simulink model "ex3"  (R2020a)
settings: Solver=VariableStepAuto  StartTime=0.0  StopTime=10.0  RelTol=1e-3
settings Model: Creator=Kundan Patil  LastModifiedBy=Kundan Patil

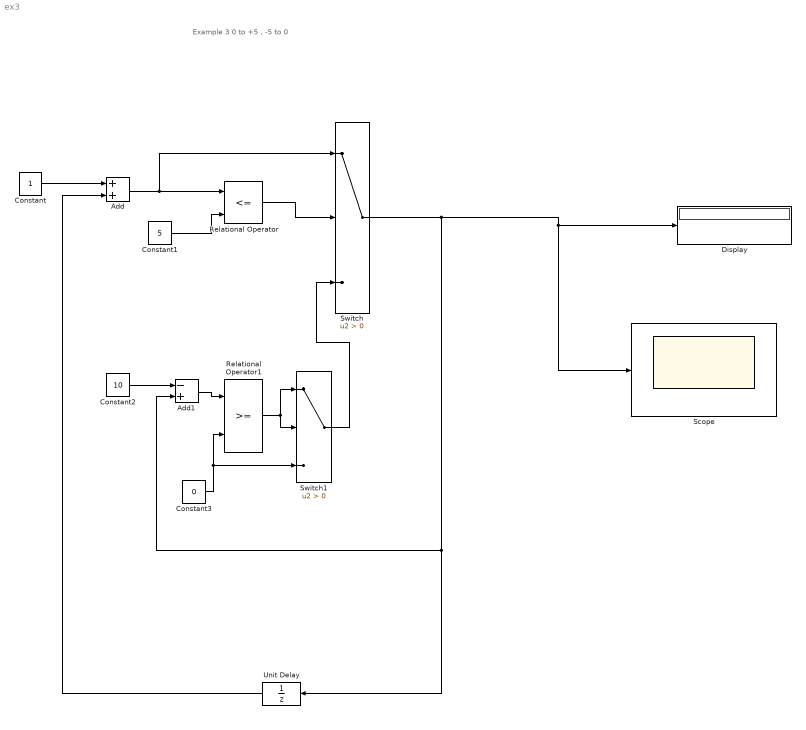
== system ex3 ==
  note: Example 3
      | 0 to +5 , -5 to 0
  Add : Sum
  Add1 : Sum  Inputs=-+
  Constant : Constant
  Constant1 : Constant  Value=5
  Constant2 : Constant  Value=10
  Constant3 : Constant  Value=0
  Display : Display
  Relational Operator : RelationalOperator  Operator=<=  OutDataTypeStr=boolean  RndMeth=Simplest
  Relational Operator1 : RelationalOperator  OutDataTypeStr=boolean  RndMeth=Simplest
  Scope : Scope
  Switch : Switch  Criteria=u2 > Threshold
  Switch1 : Switch  Criteria=u2 > Threshold
  Unit Delay : UnitDelay  InitialCondition=-1  SampleTime=-1  HasFrameUpgradeWarning=on
  wires:
  Add/1 -> Relational Operator/1, Switch/1
  Constant1/1 -> Relational Operator/2
  Switch/1 -> Scope/1, Display/1, Add1/2, Unit Delay/1
  Unit Delay/1 -> Add/2
  Constant/1 -> Add/1
  Relational Operator/1 -> Switch/2
  Constant2/1 -> Add1/1
  Add1/1 -> Relational Operator1/1
  Constant3/1 -> Switch1/3, Relational Operator1/2
  Relational Operator1/1 -> Switch1/2, Switch1/1
  Switch1/1 -> Switch/3
